simulink model "simulink_bouncingBall"  (R2018b)
settings: Solver=VariableStepAuto  StartTime=0.0  StopTime=10.0  MaxStep=0.01  RelTol=1e-3
settings Model: Creator=ak22emur  LastModifiedBy=ak22emur

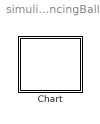
== system simulink_bouncingBall ==
  Chart : Stateflow chart  TreatAsAtomicUnit=on

== stateflow chart simulink_bouncingBall/Chart ==
  settings: updateMethod=CONTINUOUS
  state falling_down
    during:
    h_dot = v;
    v_dot = -10;
  state flying_upwards
    during:
    h_dot = v;
    v_dot = -10;
  (default) -> falling_down : {h=1; v=0;}
  falling_down -> flying_upwards : [false && h == 0]
      | {v = 0.9*v}
  flying_upwards -> falling_down : [v == 0]
  data: h local double; v local double
  data h settings: updateMethod=SF_CONTINUOUS_TIME_DATA
  data v settings: updateMethod=SF_CONTINUOUS_TIME_DATA
